simulink model "untitled1"  (R2019b)
settings: Solver=VariableStepAuto  StartTime=0.0  StopTime=1  RelTol=1e-3
settings Model: Creator=IwiLL  LastModifiedBy=IwiLL

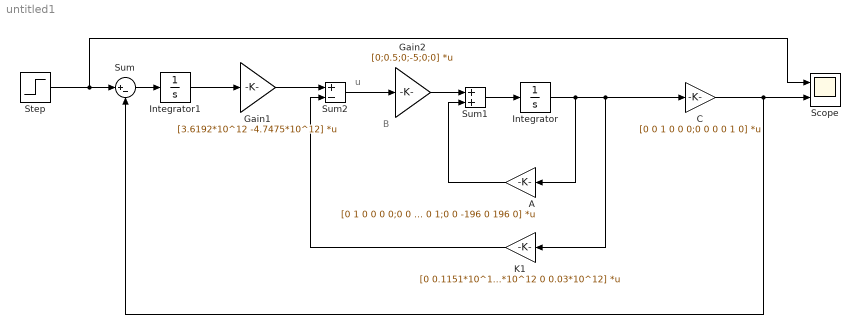
== system untitled1 ==
  note: B
  note: u
  A : Gain  Gain=[0 1 0 0 0 0;0 0 -0.98 0 0 0;0 0 0 1 0 0;0 0 205.8 0 -98 0;0 0 0 0 0 1;0 0 -196 0 196 0]  Multiplication=Matrix(K*u)
  C : Gain  Gain=[0 0 1 0 0 0;0 0 0 0 1 0]  Multiplication=Matrix(K*u)
  Gain1 : Gain  Gain=[3.6192*10^12 -4.7475*10^12]  Multiplication=Matrix(K*u)
  Gain2 : Gain  Gain=[0;0.5;0;-5;0;0]  Multiplication=Matrix(K*u)
  Integrator : Integrator  InitialCondition=rand(6,1)
  Integrator1 : Integrator
  K1 : Gain  Gain=[0 0.1151*10^12 0 0.01115*10^12 0 0.03*10^12]  Multiplication=Matrix(K*u)
  Scope : Scope  NumInputPorts=2
  Step : Step  Time=0  SampleTime=0
  Sum : Sum  Inputs=|+-
  Sum1 : Sum
  Sum2 : Sum  Inputs=+-
  wires:
  Step/1 -> Scope/1, Sum/1
  Integrator/1 -> A/1, C/1, K1/1
  Sum1/1 -> Integrator/1
  K1/1 -> Sum2/2
  Gain2/1 -> Sum1/1
  A/1 -> Sum1/2
  Sum2/1 -> Gain2/1
  C/1 -> Sum/2, Scope/2
  Gain1/1 -> Sum2/1
  Integrator1/1 -> Gain1/1
  Sum/1 -> Integrator1/1
